simulink model "DCMG_FC"  (R2022a)
settings: Solver=FixedStepAuto  StartTime=0.0  StopTime=0.2  FixedStep=Ts  MaxStep=1e-2  RelTol=1e-3
InitFcn:
  | Set_parameters_R2018
undefined symbols (not defined in the file): Ion, Lithium, R_Load_DC, Ts, Ts_Power, Vnom_DC
libraries: spsSeriesRLCBranchLib x5, spsMeanLib x5, simulink x4, spsBreakerLib x4, spsCurrentMeasurementLib x4, spsVoltageMeasurementLib x3, spsBatteryLib x1, spsControlledCurrentSourceLib x1, spsControlledVoltageSourceLib x1, spspowerguiLib x1
settings Model: Creator=Leony  LastModifiedBy=thoma
settings SolverCC: ZeroCrossAlgorithm=Adaptive  AlgebraicLoopSolver=TrustRegion  SolverResetMethod=Robust
settings DataIOCC: LimitDataPoints=on  SaveFormat=Array  ReturnWorkspaceOutputs=off
settings OptimizationCC: LifeSpan=inf
settings DebuggingCC: AlgebraicLoopMsg=none  UnderspecifiedInitializationDetection=Classic  MergeDetectMultiDrivingBlocksExec=none  IgnoredZcDiagnostic=none  SolverPrmCheckMsg=warning  UnconnectedInputMsg=warning  UnconnectedOutputMsg=warning  UnconnectedLineMsg=warning  AllowSymbolicDim=off  SFUnexpectedBacktrackingDiag=warning  SFNoUnconditionalDefaultTransitionDiag=warning  SFExecutionAtInitializationDiag=none  SFMachineParentedDataDiag=warning  ArithmeticOperatorsInVariantConditions=warning
settings HardwareCC: ProdBitPerPointer=32  ProdBitPerSizeT=32  ProdBitPerPtrDiffT=32  ProdLargestAtomicFloat=None  ProdIntDivRoundTo=Undefined  ProdEndianess=Unspecified  ProdWordSize=32  ProdHWDeviceType=32-bit Generic
settings ModelReferenceCC: PropagateSignalLabelsOutOfModel=off
settings SFSimCC: SimUseLocalCustomCode=off  CustomCodeUndefinedFunction=UseInterfaceOnly
settings RTWCC: RTWUseLocalCustomCode=off  DLArmComputeVersion=19.05
settings CodeAppCC: StateflowObjectComments=on
settings GRTTargetCC: TargetLangStandard=C89/C90 (ANSI)
settings ConfigComp: CovMetricSettings=dw  CovSaveCumulativeToWorkspaceVar=on  CovSaveSingleToWorkspaceVar=on  CovExternalEMLEnable=off
settings SimscapeCC: SimscapeNormalizeSystem=off

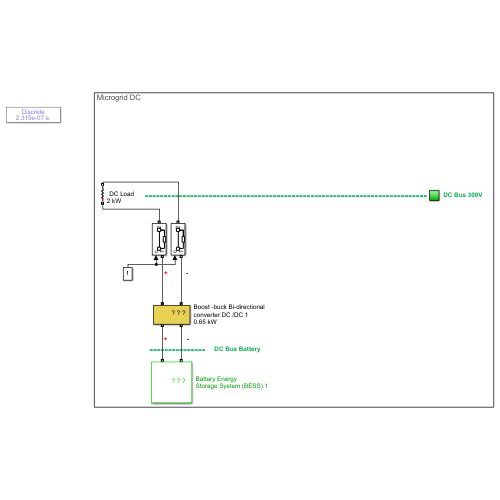
[thumbnail: Simulink's stored preview of the top-level diagram]
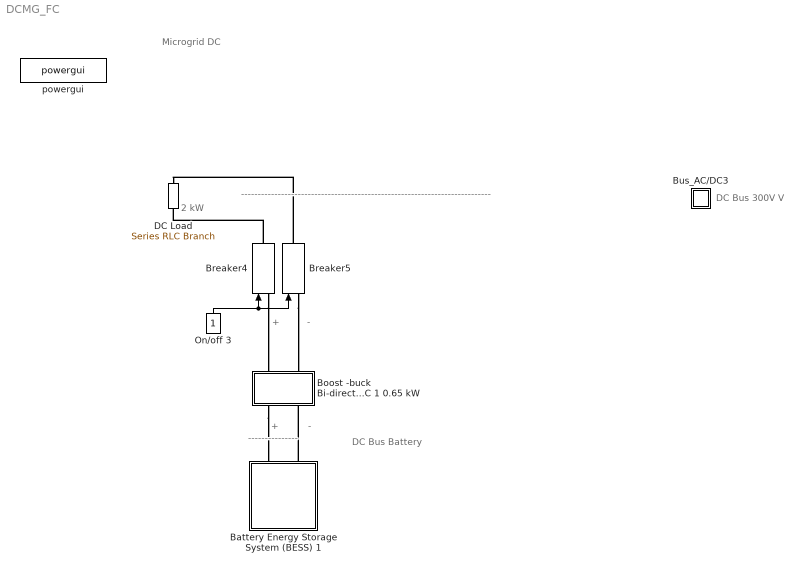
== system DCMG_FC ==
  note: ---------------------------------------------------------------------------
  note: -
  note: DC Bus Battery
  note: DC Bus 300V V
  note: +
  note: ---------------
  note: -
  note: 2 kW
  note: +
  note: Microgrid DC
  Battery Energy Storage System (BESS) 1 : Subsystem
      mask Display: image('Icons\Battery Energy Storage System (BESS).png');
  Boost -buck Bi-directional converter DC /DC 1 0.65 kW : Subsystem
      mask Display: image(imread('Icons\DC_DC_Converter.jpg'));
  Breaker4 : spsBreakerLib/Breaker  InitialState=1  SwitchingTimes="[1/60  5/60]"  External=on  BreakerResistance=0.01  SnubberResistance=1e6  SnubberCapacitance=inf  Measurements=None  MoreParameters=on  NoBreakLoop=off
      settings: SourceProductBaseCode=PS
  Breaker5 : spsBreakerLib/Breaker  InitialState=1  SwitchingTimes="[1/60  5/60]"  External=on  BreakerResistance=0.01  SnubberResistance=1e6  SnubberCapacitance=inf  Measurements=None  MoreParameters=on  NoBreakLoop=off
      settings: SourceProductBaseCode=PS
  Bus_AC/DC3 : Subsystem
  DC Load : spsSeriesRLCBranchLib/Series RLC Branch  LConnTagsString=__new0  RConnTagsString=__new0  BranchType=R  Resistance=R_Load_DC  Inductance=1e-3  SetiL0=off  InitialCurrent=0  Capacitance=1e-6  Setx0=off  InitialVoltage=0  Measurements=None
  On/off 3 : Constant
  powergui : spspowerguiLib/powergui  Priority=1  SimulationMode=Discrete  SampleTime=Ts_Power  frequency=60  Iterations=50  frequencyindice=0  Pbase=100e6  ErrMax=1e-4  UnitsV=kV  UnitsW=MW  buscounter=0  FunctionMessages=off  echomessages=off  EnableUseOfTLC=off  CurrentSourceSwitches=off  DisableSnubberDevices=off  DisableRonSwitches=off  DisableVfSwitches=off  DisplayEquations=off  AutomaticDiscreteSolvers=off  SolverType=Tustin  Interpol=off  ExternalGateDelay=off  methode=off  Ts=0  x0status=blocks  SPID=off  SwTol=0  HookPort=off  NonlinearTolerance=1e-4  nMaxIteration=100  ContinueOnMaxIteration=off  RestoreLinks=warning  ResistiveCurrentMeasurement=off  Frange=[0:2:500]  Ylog=off  Xlog=on  ShowGrid=off  save=off  variable=ZData  structure=0  ZoomFFT=off  StartTime=0.0  cycles=1  DisplayStyle=1  fundamental=60  FreqAxis=off  MaxFrequency=1000  frequencyindicesteady=1  RmsSteady=1  display=off
  wires:
  On/off 3/1 -> Breaker5/1, Breaker4/1
  connections:
  Breaker5/RConn1 -- DC Load/RConn1
  Breaker4/RConn1 -- DC Load/LConn1
  Battery Energy Storage System (BESS) 1/LConn2 -- Boost -buck Bi-directional converter DC /DC 1 0.65 kW/LConn2
  Breaker5/LConn1 -- Boost -buck Bi-directional converter DC /DC 1 0.65 kW/RConn2
  Boost -buck Bi-directional converter DC /DC 1 0.65 kW/LConn1 -- Battery Energy Storage System (BESS) 1/LConn1
  Breaker4/LConn1 -- Boost -buck Bi-directional converter DC /DC 1 0.65 kW/RConn1

== system DCMG_FC/Battery Energy Storage System (BESS) 1 ==
  Battery1 : spsBatteryLib/Battery  BatType=Lithium-Ion  ShowTempParam=off  ThermalPreset=no  ShowAgeParam=off  NomV=120  NomQ=800  SOC=80  Batt_Tr=3  PresetModel=on  MaxQ=800  MinV=90  FullV=139.6785  Dis_rate=347.8261  R=0.0015  Normal_OP=723.4783  expZone="[129.6463      39.30435]"  current=[30 35 40 46]  Units=Time  Tci=20  NomT=25  T2=0  MaxQ2=2.208  FullV2=3.45  Normal_OP2=2.8  expZone2="[3.22        0.23]"  Rca=0.6  ti=1000  Dp=0  Neq0=0  Tsim=1e6  Ta1=25  Qeol=5.4*0.9  Reol=0.013333*1.2  Char_age=[2.3478, 3]  Dis_age=[2.3478, 10]  N1=1500  N2=10500  N3=1000  N4=1400  Ta2=45  N5=950
  + B1 : PMIOPort  Side=Left
  - B1 : PMIOPort  Port=2  Side=Left
  connections:
  Battery1/LConn2 -- - B1/RConn1
  Battery1/LConn1 -- + B1/RConn1

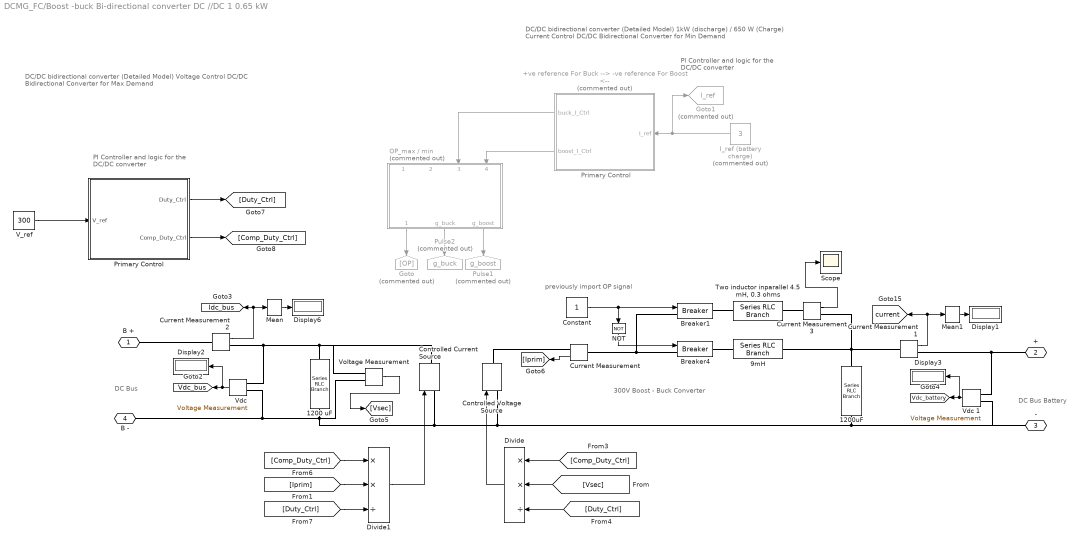
== system DCMG_FC/Boost -buck Bi-directional converter DC //DC 1 0.65 kW ==
  note: previously import OP signal
  note: Primary Control
  note: DC Bus
  note: DC Bus Battery
  note: PI Controller and logic for
      | the DC/DC converter
  note: DC/DC bidirectional converter (Detailed Model)
      | Voltage Control DC/DC Bidirectional Converter for Max Demand
  note: 300V
      | Boost - Buck Converter
  note: PI Controller and logic for
      | the DC/DC converter
  note: DC/DC bidirectional converter (Detailed Model)
      | 1kW (discharge) / 650 W (Charge)
      | Current Control DC/DC Bidirectional Converter for Min Demand
  +ve reference For Buck --> -ve reference For Boost <-- : Subsystem  Commented=on
      mask Display: image('Icons\FPGA.png');
  1200 uF : spsSeriesRLCBranchLib/Series RLC Branch  LConnTagsString=__new0  RConnTagsString=__new0  BranchType=RC  Resistance=0.1  Inductance=3e-3  SetiL0=off  InitialCurrent=0  Capacitance=120e-6  Setx0=on  InitialVoltage=300  Measurements=None
  1200uF : spsSeriesRLCBranchLib/Series RLC Branch  LConnTagsString=__new0  RConnTagsString=__new0  BranchType=C  Resistance=1  Inductance=3e-3  SetiL0=off  InitialCurrent=0  Capacitance=1200e-6  Setx0=on  InitialVoltage=120  Measurements=None
  9mH : spsSeriesRLCBranchLib/Series RLC Branch  LConnTagsString=__new0  RConnTagsString=__new0  BranchType=L  Resistance=1  Inductance=9e-3  SetiL0=off  InitialCurrent=0  Capacitance=1e-6  Setx0=off  InitialVoltage=0  Measurements=None
  Breaker1 : spsBreakerLib/Breaker  InitialState=0  SwitchingTimes="[1/60  5/60]"  External=on  BreakerResistance=0.0001  SnubberResistance=1e6  SnubberCapacitance=inf  Measurements=None  MoreParameters=on  NoBreakLoop=off
      settings: SourceProductBaseCode=PS
  Breaker4 : spsBreakerLib/Breaker  InitialState=0  SwitchingTimes="[1/60  5/60]"  External=on  BreakerResistance=0.0001  SnubberResistance=1e6  SnubberCapacitance=inf  Measurements=None  MoreParameters=on  NoBreakLoop=off
      settings: SourceProductBaseCode=PS
  Constant : Constant
  Controlled Current Source : spsControlledCurrentSourceLib/Controlled Current Source  Initialize=on  Source_Type=AC  Amplitude=0  Phase=0  Frequency=0  Measurements=None
  Controlled Voltage Source : spsControlledVoltageSourceLib/Controlled Voltage Source  Initialize=on  Source_Type=DC  Amplitude=0  Phase=0  Frequency=0  Measurements=None
  Current Measurement{,1..3} (4 alike) : spsCurrentMeasurementLib/Current Measurement  PhasorSimulation=off  OutputType=Complex  PSBequivalent=0
  Display{1..3,6} (4 alike) : Display
  Divide : Product  Inputs=**/
  Divide1 : Product  Inputs=**/
  Goto : Goto  Commented=on  GotoTag=OP
  Goto1 : Goto  Commented=on  GotoTag=I_ref  TagVisibility=global
  I_ref (battery charge) : Constant  Commented=on  Value=3
  Mean : spsMeanLib/Mean  Freq=10  Vinit=0  Ts=0
  Mean1 : spsMeanLib/Mean  Freq=10  Vinit=0  Ts=0
  NOT : Logic  Operator=NOT  IconShape=distinctive  AllPortsSameDT=off  OutDataTypeStr=boolean
  OP_max / min : Subsystem  Commented=on
  Primary Control : Subsystem
      mask Display: image('Icons\FPGA.png');
  Pulse1 : Goto  Commented=on  GotoTag=g_boost  TagVisibility=global
  Pulse2 : Goto  Commented=on  GotoTag=g_buck  TagVisibility=global
  Scope : Scope
  "Two inductor inparallel 4.5 mH, 0.3 ohms" : spsSeriesRLCBranchLib/Series RLC Branch  LConnTagsString=__new0  RConnTagsString=__new0  BranchType=RL  Resistance=0.3  Inductance=4.5e-5  SetiL0=off  InitialCurrent=0  Capacitance=1e-6  Setx0=off  InitialVoltage=0  Measurements=None
  V_ref : Constant  Value=300
  "Vdc " : spsVoltageMeasurementLib/Voltage Measurement  Tag=PoWeRsYsTeMmEaSuReMeNt  PhasorSimulation=off  OutputType=Magnitude  PSBequivalent=0
  Vdc 1 : spsVoltageMeasurementLib/Voltage Measurement  Tag=PoWeRsYsTeMmEaSuReMeNt  PhasorSimulation=off  OutputType=Magnitude  PSBequivalent=0
  Voltage Measurement : spsVoltageMeasurementLib/Voltage Measurement  PhasorSimulation=off  OutputType=Complex  PSBequivalent=0
  B + : PMIOPort  Side=Right
  + : PMIOPort  Port=2  Side=Left
  - : PMIOPort  Port=3  Side=Left
  B - : PMIOPort  Port=4  Side=Right
  tag scope: Idc_bus=global, Vdc_battery=global, Vdc_bus=global, current=global
  wires:
  "Vdc "/1 -> Display2/1, [Vdc_bus]
  Vdc 1/1 -> Display3/1, [Vdc_battery]
  Current Measurement2/1 -> Mean/1, [Idc_bus]
  Mean/1 -> Display6/1
  Current Measurement1/1 -> [current], Mean1/1
  Mean1/1 -> Display1/1
  V_ref/1 -> Primary Control/1(V_ref)
  OP_max / min/1(Op_Max / Min) -> Goto/1
  Constant/1 -> NOT/1, Breaker1/1
  NOT/1 -> Breaker4/1
  I_ref (battery charge)/1 -> Goto1/1, +ve reference For Buck --> -ve reference For Boost <--/1(I_ref)
  +ve reference For Buck --> -ve reference For Boost <--/1(buck_I_Ctrl) -> OP_max / min/3(buck_I_Ctrl)
  +ve reference For Buck --> -ve reference For Boost <--/2(boost_I_Ctrl) -> OP_max / min/4(boost_I_Ctrll)
  OP_max / min/2(g_buck) -> Pulse2/1
  OP_max / min/3(g_boost) -> Pulse1/1
  Current Measurement3/1 -> Scope/1
  Voltage Measurement/1 -> [Vsec]
  Current Measurement/1 -> [Iprim]
  Primary Control/1(Duty_Ctrl) -> [Duty_Ctrl]
  Primary Control/2(Comp_Duty_Ctrl) -> [Comp_Duty_Ctrl]
  [Vsec] -> Divide/2
  Divide/1 -> Controlled Voltage Source/1
  [Comp_Duty_Ctrl] -> Divide1/1
  [Iprim] -> Divide1/2
  [Duty_Ctrl] -> Divide1/3
  Divide1/1 -> Controlled Current Source/1
  [Comp_Duty_Ctrl] -> Divide/1
  [Duty_Ctrl] -> Divide/3
  connections:
  +/RConn1 -- Vdc 1/LConn1 -- Current Measurement1/RConn1
  Current Measurement/LConn1 -- Breaker1/LConn1 -- Breaker4/LConn1
  "Vdc "/LConn1 -- Current Measurement2/RConn1 -- 1200 uF/LConn1 -- Controlled Current Source/RConn1 -- Voltage Measurement/LConn1
  Voltage Measurement/LConn2 -- "Vdc "/LConn2 -- B -/RConn1 -- 1200 uF/RConn1 -- Controlled Voltage Source/LConn1 -- Vdc 1/LConn2 -- -/RConn1 -- 1200uF/RConn1 -- Controlled Current Source/LConn1
  Current Measurement2/LConn1 -- B +/RConn1
  "Two inductor inparallel 4.5 mH, 0.3 ohms"/LConn1 -- Breaker1/RConn1
  Current Measurement1/LConn1 -- Current Measurement3/RConn1 -- 1200uF/LConn1 -- 9mH/RConn1
  9mH/LConn1 -- Breaker4/RConn1
  "Two inductor inparallel 4.5 mH, 0.3 ohms"/RConn1 -- Current Measurement3/LConn1
  Current Measurement/RConn1 -- Controlled Voltage Source/RConn1

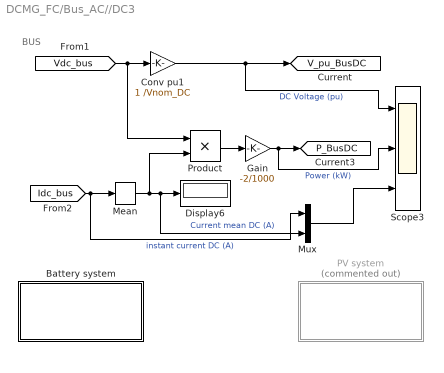
== system DCMG_FC/Bus_AC//DC3 ==
  note: BUS
  Battery system : Subsystem
      mask Display: disp('Open this block\nto display additional \nscopes & measurements')
  Conv pu1 : Gain  Gain=1 /Vnom_DC  SaturateOnIntegerOverflow=on  OutDataTypeStr=Inherit: Same as input  ParamDataTypeStr=Inherit: Same as input
  Display6 : Display
  Gain : Gain  Gain=-2/1000
  Mean : spsMeanLib/Mean  Freq=100  Vinit=0  Ts=0
  Mux : Mux  Inputs=2
  PV system : Subsystem  Commented=on
      mask Display: disp('Open this block\nto display additional \nscopes & measurements')
  Product : Product
  Scope3 : Scope  NumInputPorts=3
  tag scope: P_BusDC=global, V_pu_BusDC=global
  wires:
  Conv pu1/1 -> Scope3/1, [V_pu_BusDC]  "DC Voltage (pu)"
  [Vdc_bus] -> Product/1, Conv pu1/1
  [Idc_bus] -> Mux/1, Mean/1  "instant current DC (A)"
  Mean/1 -> Product/2, Mux/2, Display6/1  "Current mean DC (A)"
  Product/1 -> Gain/1
  Mux/1 -> Scope3/3
  Gain/1 -> Scope3/2, [P_BusDC]  "Power (kW)"

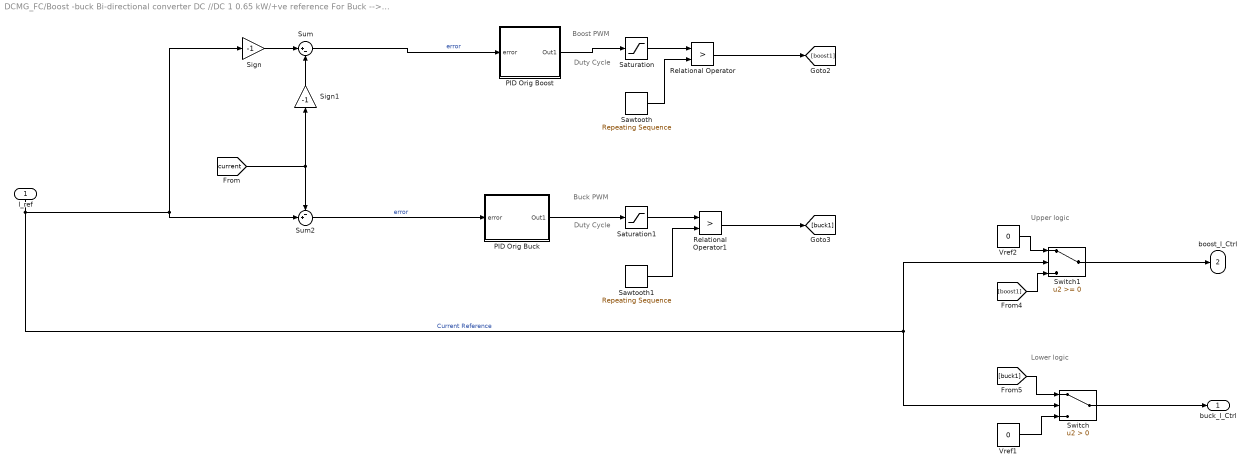
== system DCMG_FC/Boost -buck Bi-directional converter DC //DC 1 0.65 kW/+ve reference For Buck --> -ve reference For Boost <-- ==
  note: Buck PWM
  note: Duty Cycle
  note: Upper logic
  note: Lower logic
  note: Boost PWM
  note: Duty Cycle
  I_ref : Inport
  PID Orig Boost : Subsystem
  PID Orig Buck : Subsystem
  Relational Operator : RelationalOperator  Operator=>  OutDataTypeStr=boolean  InputSameDT=off
  Relational Operator1 : RelationalOperator  Operator=>  OutDataTypeStr=boolean  InputSameDT=off
  Saturation : Saturate  UpperLimit=0.9  LowerLimit=0
  Saturation1 : Saturate  UpperLimit=0.8  LowerLimit=0
  Sawtooth : simulink/Sources/Repeating Sequence  rep_seq_t=[0 1/5000]  rep_seq_y=[0 1]
  Sawtooth1 : simulink/Sources/Repeating Sequence  rep_seq_t=[0 1/5000]  rep_seq_y=[0 1]
  Sign : Gain  Gain=-1
  Sign1 : Gain  Gain=-1
  Sum : Sum  Inputs=|+-
  Sum2 : Sum  Inputs=-+|
  Switch : Switch  Criteria=u2 > Threshold  SaturateOnIntegerOverflow=off  InputSameDT=off
  Switch1 : Switch  SaturateOnIntegerOverflow=off  InputSameDT=off
  Vref1 : Constant  Value=0
  Vref2 : Constant  Value=0
  buck_I_Ctrl : Outport  VectorParamsAs1DForOutWhenUnconnected=off
  boost_I_Ctrl : Outport  Port=2  VectorParamsAs1DForOutWhenUnconnected=off
  wires:
  Sum/1 -> PID Orig Boost/1(error)  "error"
  Relational Operator/1 -> [boost1]
  Sign/1 -> Sum/1
  PID Orig Boost/1(Out1) -> Saturation/1
  PID Orig Buck/1(Out1) -> Saturation1/1
  Sawtooth/1 -> Relational Operator/2
  Sawtooth1/1 -> Relational Operator1/2
  Relational Operator1/1 -> [buck1]
  Sum2/1 -> PID Orig Buck/1(error)  "error"
  Saturation/1 -> Relational Operator/1
  Saturation1/1 -> Relational Operator1/1
  Vref1/1 -> Switch/3
  Vref2/1 -> Switch1/1
  [boost1] -> Switch1/3
  [buck1] -> Switch/1
  I_ref/1 -> Switch1/2, Switch/2, Sum2/2, Sign/1  "Current Reference"
  Sign1/1 -> Sum/2
  Switch1/1 -> boost_I_Ctrl/1
  Switch/1 -> buck_I_Ctrl/1
  [current] -> Sum2/1, Sign1/1

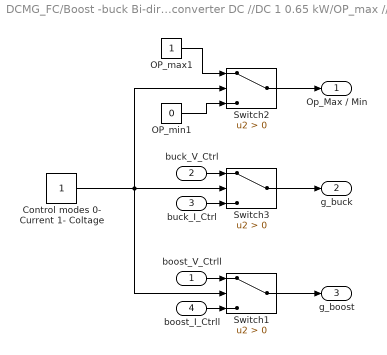
== system DCMG_FC/Boost -buck Bi-directional converter DC //DC 1 0.65 kW/OP_max // min ==
  boost_V_Ctrll : Inport
  buck_V_Ctrl : Inport  Port=2
  buck_I_Ctrl : Inport  Port=3
  boost_I_Ctrll : Inport  Port=4
  Control modes 0- Current 1- Coltage : Constant
  OP_max1 : Constant
  OP_min1 : Constant  Value=0
  Switch1 : Switch  Criteria=u2 > Threshold  SaturateOnIntegerOverflow=off  InputSameDT=off
  Switch2 : Switch  Criteria=u2 > Threshold  SaturateOnIntegerOverflow=off  InputSameDT=off
  Switch3 : Switch  Criteria=u2 > Threshold  SaturateOnIntegerOverflow=off  InputSameDT=off
  Op_Max / Min : Outport  VectorParamsAs1DForOutWhenUnconnected=off
  g_buck : Outport  Port=2  VectorParamsAs1DForOutWhenUnconnected=off
  g_boost : Outport  Port=3  VectorParamsAs1DForOutWhenUnconnected=off
  wires:
  OP_max1/1 -> Switch2/1
  OP_min1/1 -> Switch2/3
  Switch2/1 -> Op_Max / Min/1
  Control modes 0- Current 1- Coltage/1 -> Switch2/2, Switch1/2, Switch3/2
  boost_I_Ctrll/1 -> Switch1/3
  boost_V_Ctrll/1 -> Switch1/1
  buck_V_Ctrl/1 -> Switch3/1
  buck_I_Ctrl/1 -> Switch3/3
  Switch1/1 -> g_boost/1
  Switch3/1 -> g_buck/1

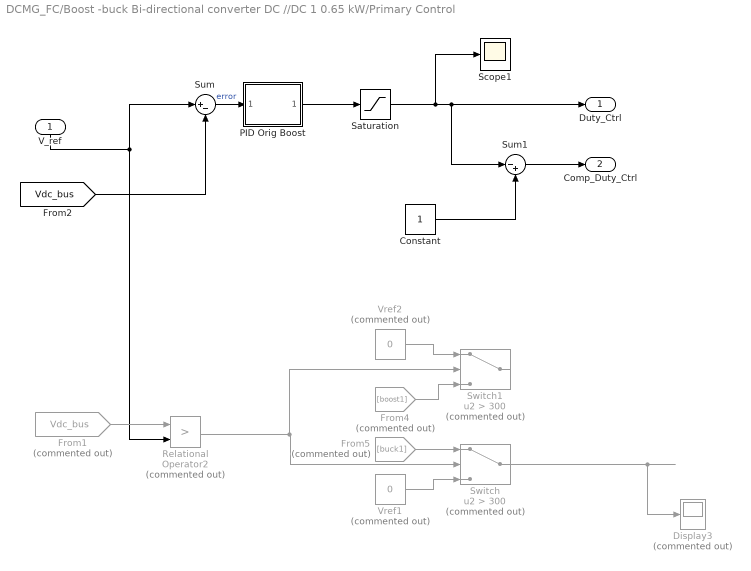
== system DCMG_FC/Boost -buck Bi-directional converter DC //DC 1 0.65 kW/Primary Control ==
  V_ref : Inport
  Constant : Constant
  Display3 : Display  Commented=on
  From1 : From  Commented=on  GotoTag=Vdc_bus  TagVisibility=global
  From4 : From  Commented=on  GotoTag=boost1
  From5 : From  Commented=on  GotoTag=buck1
  PID Orig Boost : Subsystem
  Relational Operator2 : RelationalOperator  Commented=on  Operator=>  OutDataTypeStr=boolean  InputSameDT=off
  Saturation : Saturate  UpperLimit=0.9  LowerLimit=0.1
  Scope1 : Scope
  Sum : Sum  Inputs=|+-
  Sum1 : Sum  Inputs=|-+
  Switch : Switch  Commented=on  Criteria=u2 > Threshold  Threshold=300  SaturateOnIntegerOverflow=off  InputSameDT=off
  Switch1 : Switch  Commented=on  Criteria=u2 > Threshold  Threshold=300  SaturateOnIntegerOverflow=off  InputSameDT=off
  Vref1 : Constant  Commented=on  Value=0
  Vref2 : Constant  Commented=on  Value=0
  Duty_Ctrl : Outport  VectorParamsAs1DForOutWhenUnconnected=off
  Comp_Duty_Ctrl : Outport  Port=2  VectorParamsAs1DForOutWhenUnconnected=off
  wires:
  Relational Operator2/1 -> Switch1/2, Switch/2
  V_ref/1 -> Sum/1, Relational Operator2/2
  From1/1 -> Relational Operator2/1
  Vref2/1 -> Switch1/1
  [Vdc_bus] -> Sum/2
  From5/1 -> Switch/1
  From4/1 -> Switch1/3
  Switch/1 -> Display3/1
  Vref1/1 -> Switch/3
  Sum/1 -> PID Orig Boost/1(error)  "error"
  PID Orig Boost/1(Out1) -> Saturation/1
  Constant/1 -> Sum1/2
  Saturation/1 -> Sum1/1, Duty_Ctrl/1, Scope1/1
  Sum1/1 -> Comp_Duty_Ctrl/1

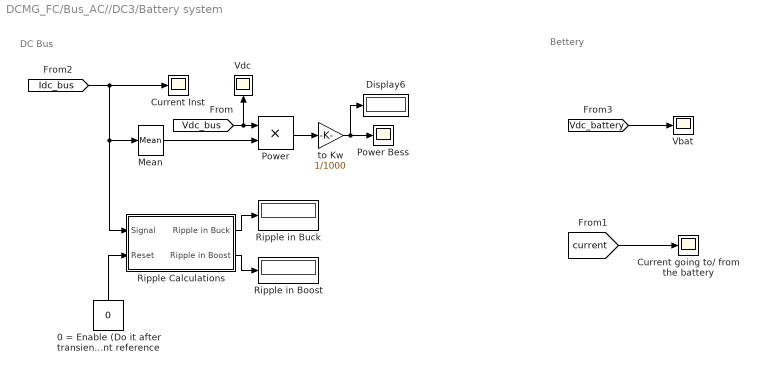
== system DCMG_FC/Bus_AC//DC3/Battery system ==
  note: DC Bus
  note: Bettery
  "0 = Enable (Do it after transient, so that it does not calculate ripples during transient) 1 = Reset after every change in current reference" : Constant  Value=0
  Current Inst : Scope
  Current going to/ from the battery : Scope
  Display6 : Display
  Mean : spsMeanLib/Mean  Freq=10  Vinit=0  Ts=0
  Power : Product
  Power Bess : Scope
  Ripple Calculations : Subsystem
  Ripple in Boost : Display
  Ripple in Buck : Display
  Vbat : Scope
  Vdc : Scope
  to Kw : Gain  Gain=1/1000
  wires:
  to Kw/1 -> Display6/1, Power Bess/1
  Mean/1 -> Power/2
  Power/1 -> to Kw/1
  Ripple Calculations/1(Ripple in Buck) -> Ripple in Buck/1
  "0 = Enable (Do it after transient, so that it does not calculate ripples during transient) 1 = Reset after every change in current reference"/1 -> Ripple Calculations/2(Reset)
  Ripple Calculations/2(Ripple in Boost) -> Ripple in Boost/1
  [Idc_bus] -> Mean/1, Ripple Calculations/1(Signal), Current Inst/1
  [current] -> Current going to/ from the battery/1
  [Vdc_bus] -> Vdc/1, Power/1
  [Vdc_battery] -> Vbat/1

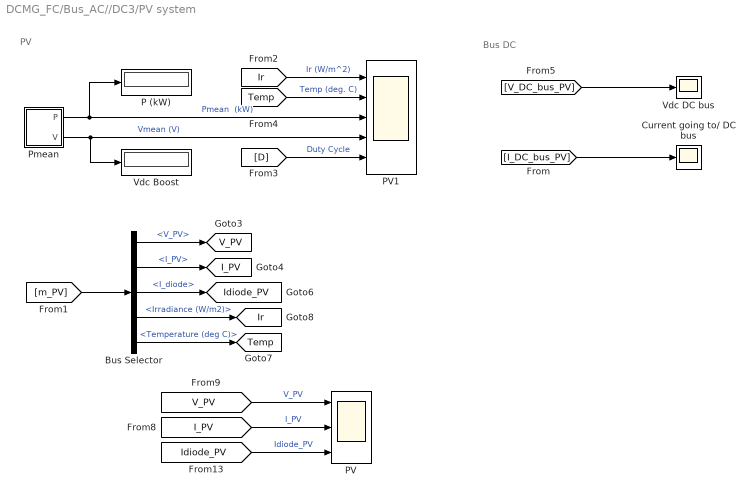
== system DCMG_FC/Bus_AC//DC3/PV system ==
  note: Bus DC
  note: PV
  Bus Selector : BusSelector  OutputSignals=V_PV,I_PV,I_diode,Irradiance (W/m2),Temperature (deg C)
  Current going to/ DC bus : Scope
  "P (kW) " : Display
      settings: Format=bank  Decimation=2000
  PV : Scope  NumInputPorts=3
  PV1 : Scope  NumInputPorts=5
  Pmean : Subsystem
  Vdc Boost : Display
      settings: Format=bank  Decimation=2000
  Vdc DC bus : Scope
  tag scope: I_PV=global, Idiode_PV=global, Ir=global, Temp=global, V_PV=global
  wires:
  [V_PV] -> PV/1  "V_PV"
  [I_PV] -> PV/2  "I_PV"
  [Idiode_PV] -> PV/3  "Idiode_PV"
  [m_PV] -> Bus Selector/1
  Bus Selector/1 -> [V_PV]  "<V_PV>"
  Bus Selector/2 -> [I_PV]  "<I_PV>"
  Bus Selector/4 -> [Ir]  "<Irradiance (W/m2)>"
  Bus Selector/3 -> [Idiode_PV]  "<I_diode>"
  Bus Selector/5 -> [Temp]  "<Temperature (deg C)>"
  [Temp] -> PV1/2  "Temp (deg. C)"
  [D] -> PV1/5  "Duty Cycle"
  Pmean/2(V) -> Vdc Boost/1, PV1/4  "Vmean (V)"
  [Ir] -> PV1/1  "Ir (W/m^2)"
  Pmean/1(P) -> "P (kW) "/1, PV1/3  "Pmean  (kW)"
  [I_DC_bus_PV] -> Current going to/ DC bus/1
  [V_DC_bus_PV] -> Vdc DC bus/1

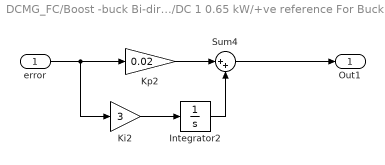
== system DCMG_FC/Boost -buck Bi-directional converter DC //DC 1 0.65 kW/+ve reference For Buck --> -ve reference For Boost <--/PID Orig Boost ==
  error : Inport
  Integrator2 : Integrator  LimitOutput=on  UpperSaturationLimit=0.9  LowerSaturationLimit=0
  Ki2 : Gain  Gain=3
  Kp2 : Gain  Gain=0.02
  Sum4 : Sum  Inputs=|++
  Out1 : Outport  VectorParamsAs1DForOutWhenUnconnected=off
  wires:
  error/1 -> Kp2/1, Ki2/1
  Kp2/1 -> Sum4/1
  Sum4/1 -> Out1/1
  Ki2/1 -> Integrator2/1
  Integrator2/1 -> Sum4/2

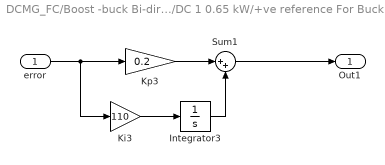
== system DCMG_FC/Boost -buck Bi-directional converter DC //DC 1 0.65 kW/+ve reference For Buck --> -ve reference For Boost <--/PID Orig Buck ==
  error : Inport
  Integrator3 : Integrator  LimitOutput=on  UpperSaturationLimit=0.9  LowerSaturationLimit=0
  Ki3 : Gain  Gain=110
  Kp3 : Gain  Gain=0.2
  Sum1 : Sum  Inputs=|++
  Out1 : Outport  VectorParamsAs1DForOutWhenUnconnected=off
  wires:
  Integrator3/1 -> Sum1/2
  Ki3/1 -> Integrator3/1
  Kp3/1 -> Sum1/1
  Sum1/1 -> Out1/1
  error/1 -> Kp3/1, Ki3/1

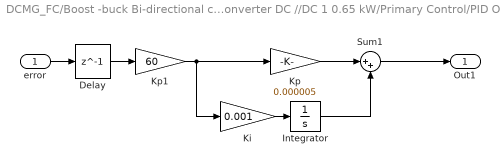
== system DCMG_FC/Boost -buck Bi-directional converter DC //DC 1 0.65 kW/Primary Control/PID Orig Boost ==
  error : Inport
  Delay : Delay  DelayLength=1  InitialCondition=0  SampleTime=Ts
  Integrator : Integrator  InitialCondition=0.1  LimitOutput=on  UpperSaturationLimit=0.9  LowerSaturationLimit=0.1
  Ki : Gain  Gain=0.001
  Kp : Gain  Gain=0.000005
  Kp1 : Gain  Gain=60
  Sum1 : Sum  Inputs=|++
  Out1 : Outport  VectorParamsAs1DForOutWhenUnconnected=off
  wires:
  Integrator/1 -> Sum1/2
  Sum1/1 -> Out1/1
  Ki/1 -> Integrator/1
  Kp/1 -> Sum1/1
  error/1 -> Delay/1
  Delay/1 -> Kp1/1
  Kp1/1 -> Kp/1, Ki/1

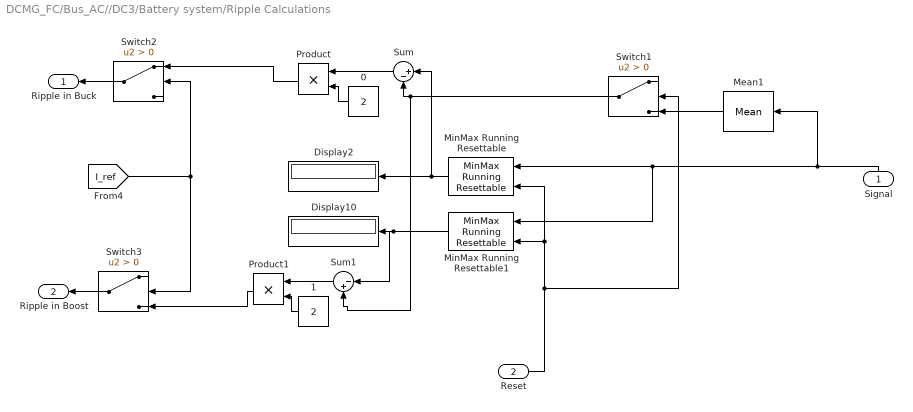
== system DCMG_FC/Bus_AC//DC3/Battery system/Ripple Calculations ==
  Signal : Inport
  Reset : Inport  Port=2
  0 : Constant  Value=2
  1 : Constant  Value=2
  Display10 : Display
  Display2 : Display
  Mean1 : spsMeanLib/Mean  Freq=10  Vinit=0  Ts=0
  MinMax Running Resettable : simulink/Math Operations/MinMax Running Resettable  Function=max  vinit=0.0
  MinMax Running Resettable1 : simulink/Math Operations/MinMax Running Resettable  Function=min  vinit=0.0
  Product : Product
  Product1 : Product
  Sum : Sum  Inputs=|+-
  Sum1 : Sum  Inputs=|-+
  Switch1 : Switch  Criteria=u2 > Threshold  SaturateOnIntegerOverflow=off  InputSameDT=off
  Switch2 : Switch  Criteria=u2 > Threshold  SaturateOnIntegerOverflow=off  InputSameDT=off
  Switch3 : Switch  Criteria=u2 > Threshold  SaturateOnIntegerOverflow=off  InputSameDT=off
  Ripple in Buck : Outport  VectorParamsAs1DForOutWhenUnconnected=off
  Ripple in Boost : Outport  Port=2  VectorParamsAs1DForOutWhenUnconnected=off
  wires:
  1/1 -> Product1/2
  [I_ref] -> Switch2/2, Switch3/2
  Product1/1 -> Switch3/3
  0/1 -> Product/2
  Switch2/1 -> Ripple in Buck/1
  Switch3/1 -> Ripple in Boost/1
  Product/1 -> Switch2/1
  Signal/1 -> Mean1/1, MinMax Running Resettable1/1, MinMax Running Resettable/1
  Switch1/1 -> Sum1/2, Sum/2
  MinMax Running Resettable/1 -> Sum/1, Display2/1
  MinMax Running Resettable1/1 -> Sum1/1, Display10/1
  Sum/1 -> Product/1
  Reset/1 -> Switch1/2, MinMax Running Resettable1/2, MinMax Running Resettable/2
  Sum1/1 -> Product1/1
  Mean1/1 -> Switch1/3

== system DCMG_FC/Bus_AC//DC3/PV system/Pmean ==
  Product : Product  RndMeth=Zero
  WkW : Gain  Gain=1/1000
  P : Outport  VectorParamsAs1DForOutWhenUnconnected=off
  V : Outport  Port=2  VectorParamsAs1DForOutWhenUnconnected=off
  wires:
  [Vmean_PV] -> Product/1, V/1
  Product/1 -> WkW/1
  [Imean_PV] -> Product/2
  WkW/1 -> P/1  "Pmean_PV (kW)"
